simulink model "idq"  (R2021a)
settings: Solver=VariableStepAuto  StartTime=0.0  StopTime=0.2  FixedStep=1/150000  MaxStep=1e-6
undefined symbols (not defined in the file): in, ou
libraries: neural x105, spsMosfetLib x12, simulink x5, pid_lib x3, spsabctodq0Lib x3, spsFirstOrderFilterLib x2, spsPermanentMagnetSynchronousMachineLib x2, spsCurrentMeasurementLib x2, spsDCVoltageSourceLib x2, spsThreePhaseVIMeasurementLib x2, spsabctoAlphaBetaZeroLib x2, spsSVPWMGenerator2LevelLib x1
(part 6 of 7)

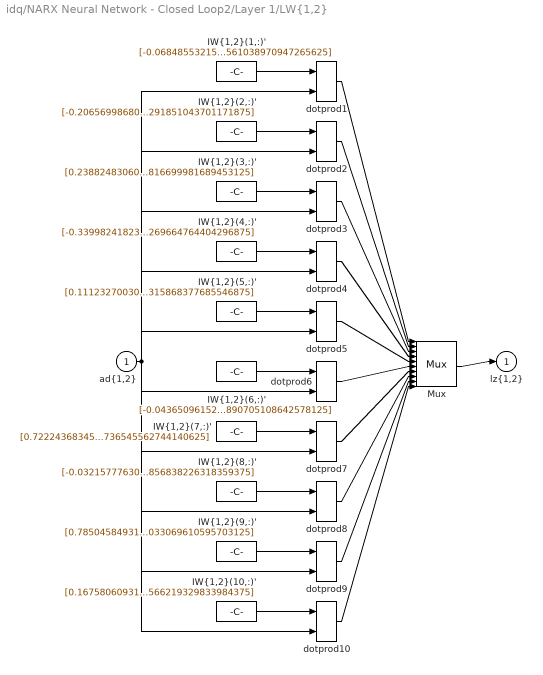
== system idq/NARX Neural Network - Closed Loop2/Layer 1/LW{1,2} ==
  "ad{1,2}" : Inport  PortDimensions=10  SampleTime=1e-05
      mask Display: e = 0.06;c1 = [120 230 180]/255;c2 = ([120 230 180]+0)/(256+128);c3 = ([120 230 180]+128)/(256+128);patch([0 1 1 0],[0 0 1 1],c1);patch([0 1 1 1-e 1-e 0+e],[0 0 1 1-e 0+e 0+e],c2);patch([0 0 1 1-e 0+e 0+e],[0 1 1 1-e 1-e 0+e],c3);plot([0 1 1 0 0],[0 0 1 1 0]);
  "IW{1,2}(1,:)'" : Constant  Value=[-0.06848553215792078929791131258753011934459209442138671875;-0.168183592807916448830241051837219856679439544677734375;-0.0232648098321999417803507270718910149298608303070068359375;0.0222599968251831863141898537605811725370585918426513671875;0.1559933939712914441333424520053085871040821075439453125;0.1043118802673528022761928468753467313945293426513671875;-0.10830870825632206433386528487972100265324115753173828125;-0.06587364865356681864483334720716811716556549072265625;0.1045799553153159144880390840626205317676067352294921875;-0.0238569322650025207599444598827176378108561038970947265625]
      mask Display: e = 0.06;c1 = [120 150 230]/255;c2 = ([120 150 230]+0)/383;c3 = ([120 150 230]+128)/383;patch([0 1 1 0],[0 0 1 1],c1);patch([0 1 1 1-e 1-e 0+e],[0 0 1 1-e 0+e 0+e],c2);patch([0 0 1 1-e 0+e 0+e],[0 1 1 1-e 1-e 0+e],c3);plot([0 1 1 0 0],[0 0 1 1 0]);disp('weights');
  "IW{1,2}(10,:)'" : Constant  Value=[0.167580609319410267499250721812131814658641815185546875;-0.033693308851453822316823760729675996117293834686279296875;-0.02316251894436265057475310413792612962424755096435546875;-0.1505391673267879870667940167550113983452320098876953125;0.0771320191346646921726204482183675281703472137451171875;-0.01480470085334451534053723520401035784743726253509521484375;0.01030379682128204459068410159261475200764834880828857421875;0.0170955227174202674389480449690381647087633609771728515625;-0.1803345239355904905398375603908789344131946563720703125;0.1414515538710732212024367981939576566219329833984375]
      mask Display: e = 0.06;c1 = [120 150 230]/255;c2 = ([120 150 230]+0)/383;c3 = ([120 150 230]+128)/383;patch([0 1 1 0],[0 0 1 1],c1);patch([0 1 1 1-e 1-e 0+e],[0 0 1 1-e 0+e 0+e],c2);patch([0 0 1 1-e 0+e 0+e],[0 1 1 1-e 1-e 0+e],c3);plot([0 1 1 0 0],[0 0 1 1 0]);disp('weights');
  "IW{1,2}(2,:)'" : Constant  Value=[-0.206569986808232075592428600430139340460300445556640625;-0.17704285291305799088235062299645505845546722412109375;0.067029514515075272473865197753184475004673004150390625;-0.11298701828022028603726312212529592216014862060546875;0.44502267784332227851251673200749792158603668212890625;0.0635628244876923209627506139440811239182949066162109375;-0.31596978877279990882698257337324321269989013671875;-0.159523136450386238127663318664417602121829986572265625;-0.026269199652980655679268551239147200249135494232177734375;0.193965717402612980446718893290380947291851043701171875]
      mask Display: e = 0.06;c1 = [120 150 230]/255;c2 = ([120 150 230]+0)/383;c3 = ([120 150 230]+128)/383;patch([0 1 1 0],[0 0 1 1],c1);patch([0 1 1 1-e 1-e 0+e],[0 0 1 1-e 0+e 0+e],c2);patch([0 0 1 1-e 0+e 0+e],[0 1 1 1-e 1-e 0+e],c3);plot([0 1 1 0 0],[0 0 1 1 0]);disp('weights');
  "IW{1,2}(3,:)'" : Constant  Value=[0.2388248306077005722602990545055945403873920440673828125;-0.022260383608824006740345424759652814827859401702880859375;-0.11939523610495351990667955988101311959326267242431640625;-0.1639270891371009952752757499183644540607929229736328125;0.39292260806126522165726555613218806684017181396484375;0.13655922559615196743010301361209712922573089599609375;-0.20158757850580144577179453335702419281005859375;-0.2125949397905498583494221520595601759850978851318359375;0.214255988741538339059644613371347077190876007080078125;0.0736149453097654504762914484672364778816699981689453125]
      mask Display: e = 0.06;c1 = [120 150 230]/255;c2 = ([120 150 230]+0)/383;c3 = ([120 150 230]+128)/383;patch([0 1 1 0],[0 0 1 1],c1);patch([0 1 1 1-e 1-e 0+e],[0 0 1 1-e 0+e 0+e],c2);patch([0 0 1 1-e 0+e 0+e],[0 1 1 1-e 1-e 0+e],c3);plot([0 1 1 0 0],[0 0 1 1 0]);disp('weights');
  "IW{1,2}(4,:)'" : Constant  Value=[-0.339982418230844685158587026307941414415836334228515625;0.06286791591134743839575094170868396759033203125;0.042782434851617374971244345260856789536774158477783203125;0.61568812941807304905950104512157849967479705810546875;-0.484514132046519330199174646622850559651851654052734375;-0.0970863636307574273676124221310601569712162017822265625;0.1572777042332852148742716735796420834958553314208984375;0.20099707904543751002535145744332112371921539306640625;0.235554356615042037592644419419229961931705474853515625;-0.3985764861287808269452170861768536269664764404296875]
      mask Display: e = 0.06;c1 = [120 150 230]/255;c2 = ([120 150 230]+0)/383;c3 = ([120 150 230]+128)/383;patch([0 1 1 0],[0 0 1 1],c1);patch([0 1 1 1-e 1-e 0+e],[0 0 1 1-e 0+e 0+e],c2);patch([0 0 1 1-e 0+e 0+e],[0 1 1 1-e 1-e 0+e],c3);plot([0 1 1 0 0],[0 0 1 1 0]);disp('weights');
  "IW{1,2}(5,:)'" : Constant  Value=[0.11123270030713751366224784078440279699862003326416015625;0.0441165371646720372300620738315046764910221099853515625;0.0337872497512030356414669540754402987658977508544921875;-0.1605454306752725213147670046964776702225208282470703125;0.0023510123039627607577362056190395378507673740386962890625;0.0243052304300900023914522307677543722093105316162109375;0.025135399965839778924081571176429861225187778472900390625;-0.02490004066075475475106060230245930142700672149658203125;-0.03397034171832931381818099225711193867027759552001953125;0.09640861696046380824309807167082908563315868377685546875]
      mask Display: e = 0.06;c1 = [120 150 230]/255;c2 = ([120 150 230]+0)/383;c3 = ([120 150 230]+128)/383;patch([0 1 1 0],[0 0 1 1],c1);patch([0 1 1 1-e 1-e 0+e],[0 0 1 1-e 0+e 0+e],c2);patch([0 0 1 1-e 0+e 0+e],[0 1 1 1-e 1-e 0+e],c3);plot([0 1 1 0 0],[0 0 1 1 0]);disp('weights');
  "IW{1,2}(6,:)'" : Constant  Value=[-0.043650961523407139086572215092019177973270416259765625;-0.0310808465779854707633500510155499796383082866668701171875;0.020776758678725339157811191626024083234369754791259765625;0.00987290351155388490322906136498204432427883148193359375;0.033604488073563969219303970703549566678702831268310546875;-0.05455938140951634152120419685161323286592960357666015625;-0.0510714350539601957823521161117241717875003814697265625;0.045197639986406086543002658117984537966549396514892578125;-0.0495999610894839182417825895754504017531871795654296875;-0.007247288368574862638116229618390207178890705108642578125]
      mask Display: e = 0.06;c1 = [120 150 230]/255;c2 = ([120 150 230]+0)/383;c3 = ([120 150 230]+128)/383;patch([0 1 1 0],[0 0 1 1],c1);patch([0 1 1 1-e 1-e 0+e],[0 0 1 1-e 0+e 0+e],c2);patch([0 0 1 1-e 0+e 0+e],[0 1 1 1-e 1-e 0+e],c3);plot([0 1 1 0 0],[0 0 1 1 0]);disp('weights');
  "IW{1,2}(7,:)'" : Constant  Value=[0.72224368345128520108033853830420412123203277587890625;-0.29672427963986247601013701569172553718090057373046875;-0.5219792424542266662257361531374044716358184814453125;-0.35115714045900736639538308736518956720829010009765625;0.40301906060842485057804651660262607038021087646484375;0.10200757360121469330405119535498670302331447601318359375;-0.03903474384426190713082149841284262947738170623779296875;0.0407956879638946556809742105542682111263275146484375;0.27212331081209339966875404570600949227809906005859375;0.120339102854654600438522038530209101736545562744140625]
      mask Display: e = 0.06;c1 = [120 150 230]/255;c2 = ([120 150 230]+0)/383;c3 = ([120 150 230]+128)/383;patch([0 1 1 0],[0 0 1 1],c1);patch([0 1 1 1-e 1-e 0+e],[0 0 1 1-e 0+e 0+e],c2);patch([0 0 1 1-e 0+e 0+e],[0 1 1 1-e 1-e 0+e],c3);plot([0 1 1 0 0],[0 0 1 1 0]);disp('weights');
  "IW{1,2}(8,:)'" : Constant  Value=[-0.03215777630550940846543284123981720767915248870849609375;-0.15179539790991791736729510375880636274814605712890625;0.044477295640847402946604915996431373059749603271484375;-0.383254418254840578672570927665219642221927642822265625;0.555254658952926138937300493125803768634796142578125;0.4168867115597614247946012255852110683917999267578125;-0.2437911984166573342580619510044925846159458160400390625;-0.6246901165206126815832021748065017163753509521484375;0.72781955521921093410497860531904734671115875244140625;-0.007339261862083799881073531423680833540856838226318359375]
      mask Display: e = 0.06;c1 = [120 150 230]/255;c2 = ([120 150 230]+0)/383;c3 = ([120 150 230]+128)/383;patch([0 1 1 0],[0 0 1 1],c1);patch([0 1 1 1-e 1-e 0+e],[0 0 1 1-e 0+e 0+e],c2);patch([0 0 1 1-e 0+e 0+e],[0 1 1 1-e 1-e 0+e],c3);plot([0 1 1 0 0],[0 0 1 1 0]);disp('weights');
  "IW{1,2}(9,:)'" : Constant  Value=[0.78504584931199727915185349047533236443996429443359375;0.252420705465960681923576203189441002905368804931640625;-0.446249033364787661692929532364360056817531585693359375;0.006236623888100943646772833517388789914548397064208984375;-0.229719455430527019768049967751721851527690887451171875;0.132202063827780824656343838796601630747318267822265625;0.186514759811286179314038236043415963649749755859375;0.1583920339325100845595528653575456701219081878662109375;0.418456055887584332797501929235295392572879791259765625;-0.399445269839285910240533894466352649033069610595703125]
      mask Display: e = 0.06;c1 = [120 150 230]/255;c2 = ([120 150 230]+0)/383;c3 = ([120 150 230]+128)/383;patch([0 1 1 0],[0 0 1 1],c1);patch([0 1 1 1-e 1-e 0+e],[0 0 1 1-e 0+e 0+e],c2);patch([0 0 1 1-e 0+e 0+e],[0 1 1 1-e 1-e 0+e],c3);plot([0 1 1 0 0],[0 0 1 1 0]);disp('weights');
  Mux : Mux  Inputs=10
      mask Display: e = 0.06;c1 = [120 150 230]/255;c2 = ([120 150 230]+0)/383;c3 = ([120 150 230]+128)/383;patch([0 1 1 0],[0 0 1 1],c1);patch([0 1 1 1-e 1-e 0+e],[0 0 1 1-e 0+e 0+e],c2);patch([0 0 1 1-e 0+e 0+e],[0 1 1 1-e 1-e 0+e],c3);plot([0 1 1 0 0],[0 0 1 1 0]);disp('Mux');
  dotprod{1..10} (10 alike) : neural/Weight Functions/dotprod
  "lz{1,2}" : Outport
      mask Display: e = 0.06;c1 = [120 230 180]/255;c2 = ([120 230 180]+0)/(256+128);c3 = ([120 230 180]+128)/(256+128);patch([0 1 1 0],[0 0 1 1],c1);patch([0 1 1 1-e 1-e 0+e],[0 0 1 1-e 0+e 0+e],c2);patch([0 0 1 1-e 0+e 0+e],[0 1 1 1-e 1-e 0+e],c3);plot([0 1 1 0 0],[0 0 1 1 0]);
  wires:
  "IW{1,2}(1,:)'"/1 -> dotprod1/1
  "ad{1,2}"/1 -> dotprod1/2, dotprod2/2, dotprod3/2, dotprod4/2, dotprod5/2, dotprod6/2, dotprod7/2, dotprod8/2, dotprod9/2, dotprod10/2
  dotprod1/1 -> Mux/1
  "IW{1,2}(2,:)'"/1 -> dotprod2/1
  dotprod2/1 -> Mux/2
  "IW{1,2}(3,:)'"/1 -> dotprod3/1
  dotprod3/1 -> Mux/3
  "IW{1,2}(4,:)'"/1 -> dotprod4/1
  dotprod4/1 -> Mux/4
  "IW{1,2}(5,:)'"/1 -> dotprod5/1
  dotprod5/1 -> Mux/5
  "IW{1,2}(6,:)'"/1 -> dotprod6/1
  dotprod6/1 -> Mux/6
  "IW{1,2}(7,:)'"/1 -> dotprod7/1
  dotprod7/1 -> Mux/7
  "IW{1,2}(8,:)'"/1 -> dotprod8/1
  dotprod8/1 -> Mux/8
  "IW{1,2}(9,:)'"/1 -> dotprod9/1
  dotprod9/1 -> Mux/9
  "IW{1,2}(10,:)'"/1 -> dotprod10/1
  dotprod10/1 -> Mux/10
  Mux/1 -> "lz{1,2}"/1

== system idq/NARX Neural Network - Closed Loop2/Layer 2/Delays 1 ==
  "p{2}" : Inport  PortDimensions=10  SampleTime=1e-05
      mask Display: e = 0.06;c1 = [120 230 180]/255;c2 = ([120 230 180]+0)/(256+128);c3 = ([120 230 180]+128)/(256+128);patch([0 1 1 0],[0 0 1 1],c1);patch([0 1 1 1-e 1-e 0+e],[0 0 1 1-e 0+e 0+e],c2);patch([0 0 1 1-e 0+e 0+e],[0 1 1 1-e 1-e 0+e],c3);plot([0 1 1 0 0],[0 0 1 1 0]);
  mux : Mux  Inputs=1
      mask Display: e = 0.06;c1 = [120 150 230]/255;c2 = ([120 150 230]+0)/383;c3 = ([120 150 230]+128)/383;patch([0 1 1 0],[0 0 1 1],c1);patch([0 1 1 1-e 1-e 0+e],[0 0 1 1-e 0+e 0+e],c2);patch([0 0 1 1-e 0+e 0+e],[0 1 1 1-e 1-e 0+e],c3);plot([0 1 1 0 0],[0 0 1 1 0]);disp('Mux')
  "pd{2,1}" : Outport
      mask Display: e = 0.06;c1 = [120 230 180]/255;c2 = ([120 230 180]+0)/(256+128);c3 = ([120 230 180]+128)/(256+128);patch([0 1 1 0],[0 0 1 1],c1);patch([0 1 1 1-e 1-e 0+e],[0 0 1 1-e 0+e 0+e],c2);patch([0 0 1 1-e 0+e 0+e],[0 1 1 1-e 1-e 0+e],c3);plot([0 1 1 0 0],[0 0 1 1 0]);
  wires:
  "p{2}"/1 -> mux/1
  mux/1 -> "pd{2,1}"/1

== system idq/NARX Neural Network - Closed Loop2/Layer 2/LW{2,1} ==
  "ad{2,1}" : Inport  PortDimensions=10  SampleTime=1e-05
      mask Display: e = 0.06;c1 = [120 230 180]/255;c2 = ([120 230 180]+0)/(256+128);c3 = ([120 230 180]+128)/(256+128);patch([0 1 1 0],[0 0 1 1],c1);patch([0 1 1 1-e 1-e 0+e],[0 0 1 1-e 0+e 0+e],c2);patch([0 0 1 1-e 0+e 0+e],[0 1 1 1-e 1-e 0+e],c3);plot([0 1 1 0 0],[0 0 1 1 0]);
  "IW{2,1}(1,:)'" : Constant  Value=[-1.8024487538491762439463172995601780712604522705078125;1.7858415231748401286182570402161218225955963134765625;-1.0516660228917158459438496720395050942897796630859375;-1.321897069778581457200061777257360517978668212890625;2.196982273081371506151526773464865982532501220703125;1.3943035974706512458709539714618586003780364990234375;-0.9205379723976834238641231422661803662776947021484375;1.012472143579025374293678396497853100299835205078125;1.0636810315768301382632898821611888706684112548828125;-2.066348426610085997623400544398464262485504150390625]
      mask Display: e = 0.06;c1 = [120 150 230]/255;c2 = ([120 150 230]+0)/383;c3 = ([120 150 230]+128)/383;patch([0 1 1 0],[0 0 1 1],c1);patch([0 1 1 1-e 1-e 0+e],[0 0 1 1-e 0+e 0+e],c2);patch([0 0 1 1-e 0+e 0+e],[0 1 1 1-e 1-e 0+e],c3);plot([0 1 1 0 0],[0 0 1 1 0]);disp('weights');
  Mux : Mux  Inputs=1
      mask Display: e = 0.06;c1 = [120 150 230]/255;c2 = ([120 150 230]+0)/383;c3 = ([120 150 230]+128)/383;patch([0 1 1 0],[0 0 1 1],c1);patch([0 1 1 1-e 1-e 0+e],[0 0 1 1-e 0+e 0+e],c2);patch([0 0 1 1-e 0+e 0+e],[0 1 1 1-e 1-e 0+e],c3);plot([0 1 1 0 0],[0 0 1 1 0]);disp('Mux');
  dotprod1 : neural/Weight Functions/dotprod
  "lz{2,1}" : Outport
      mask Display: e = 0.06;c1 = [120 230 180]/255;c2 = ([120 230 180]+0)/(256+128);c3 = ([120 230 180]+128)/(256+128);patch([0 1 1 0],[0 0 1 1],c1);patch([0 1 1 1-e 1-e 0+e],[0 0 1 1-e 0+e 0+e],c2);patch([0 0 1 1-e 0+e 0+e],[0 1 1 1-e 1-e 0+e],c3);plot([0 1 1 0 0],[0 0 1 1 0]);
  wires:
  "IW{2,1}(1,:)'"/1 -> dotprod1/1
  "ad{2,1}"/1 -> dotprod1/2
  dotprod1/1 -> Mux/1
  Mux/1 -> "lz{2,1}"/1

== system idq/Time Delay Neural Network1/Layer 1/Delays 1 ==
  "p{1}" : Inport  PortDimensions=4  SampleTime=1e-05
      mask Display: e = 0.06;c1 = [120 230 180]/255;c2 = ([120 230 180]+0)/(256+128);c3 = ([120 230 180]+128)/(256+128);patch([0 1 1 0],[0 0 1 1],c1);patch([0 1 1 1-e 1-e 0+e],[0 0 1 1-e 0+e 0+e],c2);patch([0 0 1 1-e 0+e 0+e],[0 1 1 1-e 1-e 0+e],c3);plot([0 1 1 0 0],[0 0 1 1 0]);
  Delay 1 : UnitDelay  InitialCondition=pi_input_1_delayed_1  SampleTime=1e-05
      mask Display: e = 0.06;c1 = [120 150 230]/255;c2 = ([120 150 230]+0)/383;c3 = ([120 150 230]+128)/383;patch([0 1 1 0],[0 0 1 1],c1);patch([0 1 1 1-e 1-e 0+e],[0 0 1 1-e 0+e 0+e],c2);patch([0 0 1 1-e 0+e 0+e],[0 1 1 1-e 1-e 0+e],c3);plot([0 1 1 0 0],[0 0 1 1 0]);disp('D')
  Delay 10 : UnitDelay  InitialCondition=pi_input_1_delayed_10  SampleTime=1e-05
      mask Display: e = 0.06;c1 = [120 150 230]/255;c2 = ([120 150 230]+0)/383;c3 = ([120 150 230]+128)/383;patch([0 1 1 0],[0 0 1 1],c1);patch([0 1 1 1-e 1-e 0+e],[0 0 1 1-e 0+e 0+e],c2);patch([0 0 1 1-e 0+e 0+e],[0 1 1 1-e 1-e 0+e],c3);plot([0 1 1 0 0],[0 0 1 1 0]);disp('D')
  Delay 2 : UnitDelay  InitialCondition=pi_input_1_delayed_2  SampleTime=1e-05
      mask Display: e = 0.06;c1 = [120 150 230]/255;c2 = ([120 150 230]+0)/383;c3 = ([120 150 230]+128)/383;patch([0 1 1 0],[0 0 1 1],c1);patch([0 1 1 1-e 1-e 0+e],[0 0 1 1-e 0+e 0+e],c2);patch([0 0 1 1-e 0+e 0+e],[0 1 1 1-e 1-e 0+e],c3);plot([0 1 1 0 0],[0 0 1 1 0]);disp('D')
  Delay 3 : UnitDelay  InitialCondition=pi_input_1_delayed_3  SampleTime=1e-05
      mask Display: e = 0.06;c1 = [120 150 230]/255;c2 = ([120 150 230]+0)/383;c3 = ([120 150 230]+128)/383;patch([0 1 1 0],[0 0 1 1],c1);patch([0 1 1 1-e 1-e 0+e],[0 0 1 1-e 0+e 0+e],c2);patch([0 0 1 1-e 0+e 0+e],[0 1 1 1-e 1-e 0+e],c3);plot([0 1 1 0 0],[0 0 1 1 0]);disp('D')
  Delay 4 : UnitDelay  InitialCondition=pi_input_1_delayed_4  SampleTime=1e-05
      mask Display: e = 0.06;c1 = [120 150 230]/255;c2 = ([120 150 230]+0)/383;c3 = ([120 150 230]+128)/383;patch([0 1 1 0],[0 0 1 1],c1);patch([0 1 1 1-e 1-e 0+e],[0 0 1 1-e 0+e 0+e],c2);patch([0 0 1 1-e 0+e 0+e],[0 1 1 1-e 1-e 0+e],c3);plot([0 1 1 0 0],[0 0 1 1 0]);disp('D')
  Delay 5 : UnitDelay  InitialCondition=pi_input_1_delayed_5  SampleTime=1e-05
      mask Display: e = 0.06;c1 = [120 150 230]/255;c2 = ([120 150 230]+0)/383;c3 = ([120 150 230]+128)/383;patch([0 1 1 0],[0 0 1 1],c1);patch([0 1 1 1-e 1-e 0+e],[0 0 1 1-e 0+e 0+e],c2);patch([0 0 1 1-e 0+e 0+e],[0 1 1 1-e 1-e 0+e],c3);plot([0 1 1 0 0],[0 0 1 1 0]);disp('D')
  Delay 6 : UnitDelay  InitialCondition=pi_input_1_delayed_6  SampleTime=1e-05
      mask Display: e = 0.06;c1 = [120 150 230]/255;c2 = ([120 150 230]+0)/383;c3 = ([120 150 230]+128)/383;patch([0 1 1 0],[0 0 1 1],c1);patch([0 1 1 1-e 1-e 0+e],[0 0 1 1-e 0+e 0+e],c2);patch([0 0 1 1-e 0+e 0+e],[0 1 1 1-e 1-e 0+e],c3);plot([0 1 1 0 0],[0 0 1 1 0]);disp('D')
  Delay 7 : UnitDelay  InitialCondition=pi_input_1_delayed_7  SampleTime=1e-05
      mask Display: e = 0.06;c1 = [120 150 230]/255;c2 = ([120 150 230]+0)/383;c3 = ([120 150 230]+128)/383;patch([0 1 1 0],[0 0 1 1],c1);patch([0 1 1 1-e 1-e 0+e],[0 0 1 1-e 0+e 0+e],c2);patch([0 0 1 1-e 0+e 0+e],[0 1 1 1-e 1-e 0+e],c3);plot([0 1 1 0 0],[0 0 1 1 0]);disp('D')
  Delay 8 : UnitDelay  InitialCondition=pi_input_1_delayed_8  SampleTime=1e-05
      mask Display: e = 0.06;c1 = [120 150 230]/255;c2 = ([120 150 230]+0)/383;c3 = ([120 150 230]+128)/383;patch([0 1 1 0],[0 0 1 1],c1);patch([0 1 1 1-e 1-e 0+e],[0 0 1 1-e 0+e 0+e],c2);patch([0 0 1 1-e 0+e 0+e],[0 1 1 1-e 1-e 0+e],c3);plot([0 1 1 0 0],[0 0 1 1 0]);disp('D')
  Delay 9 : UnitDelay  InitialCondition=pi_input_1_delayed_9  SampleTime=1e-05
      mask Display: e = 0.06;c1 = [120 150 230]/255;c2 = ([120 150 230]+0)/383;c3 = ([120 150 230]+128)/383;patch([0 1 1 0],[0 0 1 1],c1);patch([0 1 1 1-e 1-e 0+e],[0 0 1 1-e 0+e 0+e],c2);patch([0 0 1 1-e 0+e 0+e],[0 1 1 1-e 1-e 0+e],c3);plot([0 1 1 0 0],[0 0 1 1 0]);disp('D')
  mux : Mux  Inputs=10
      mask Display: e = 0.06;c1 = [120 150 230]/255;c2 = ([120 150 230]+0)/383;c3 = ([120 150 230]+128)/383;patch([0 1 1 0],[0 0 1 1],c1);patch([0 1 1 1-e 1-e 0+e],[0 0 1 1-e 0+e 0+e],c2);patch([0 0 1 1-e 0+e 0+e],[0 1 1 1-e 1-e 0+e],c3);plot([0 1 1 0 0],[0 0 1 1 0]);disp('Mux')
  "pd{1,1}" : Outport
      mask Display: e = 0.06;c1 = [120 230 180]/255;c2 = ([120 230 180]+0)/(256+128);c3 = ([120 230 180]+128)/(256+128);patch([0 1 1 0],[0 0 1 1],c1);patch([0 1 1 1-e 1-e 0+e],[0 0 1 1-e 0+e 0+e],c2);patch([0 0 1 1-e 0+e 0+e],[0 1 1 1-e 1-e 0+e],c3);plot([0 1 1 0 0],[0 0 1 1 0]);
  wires:
  "p{1}"/1 -> Delay 1/1
  Delay 1/1 -> Delay 2/1, mux/1
  Delay 2/1 -> Delay 3/1, mux/2
  Delay 3/1 -> Delay 4/1, mux/3
  Delay 4/1 -> Delay 5/1, mux/4
  Delay 5/1 -> Delay 6/1, mux/5
  Delay 6/1 -> Delay 7/1, mux/6
  Delay 7/1 -> Delay 8/1, mux/7
  Delay 8/1 -> Delay 9/1, mux/8
  Delay 9/1 -> Delay 10/1, mux/9
  Delay 10/1 -> mux/10
  mux/1 -> "pd{1,1}"/1

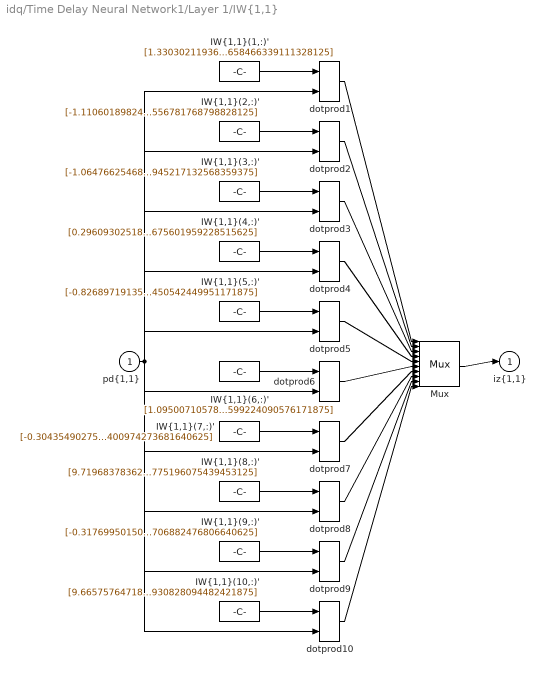
== system idq/Time Delay Neural Network1/Layer 1/IW{1,1} ==
  "pd{1,1}" : Inport  PortDimensions=40  SampleTime=1e-05
      mask Display: e = 0.06;c1 = [120 230 180]/255;c2 = ([120 230 180]+0)/(256+128);c3 = ([120 230 180]+128)/(256+128);patch([0 1 1 0],[0 0 1 1],c1);patch([0 1 1 1-e 1-e 0+e],[0 0 1 1-e 0+e 0+e],c2);patch([0 0 1 1-e 0+e 0+e],[0 1 1 1-e 1-e 0+e],c3);plot([0 1 1 0 0],[0 0 1 1 0]);
  "IW{1,1}(1,:)'" : Constant  Value=[1.330302119368188318304646600154228508472442626953125;0.0926808503977066544532448233439936302602291107177734375;-11.289158332529421358003673958592116832733154296875;10.5997790536904705760434808325953781604766845703125;-0.139965464238469505797723968498758040368556976318359375;-0.93598840560570495394898671293049119412899017333984375;-8.4957112256748370526793223689310252666473388671875;7.4618720824951143555381349870003759860992431640625;2.29448920327525396345436092815361917018890380859375;0.1828678635635263283187867955348338000476360321044921875;-6.07154144858802879980430589057505130767822265625;4.4847061641032386347660576575435698032379150390625;1.1386507448784135565489350483403541147708892822265625;-1.3104699105953994120454808580689132213592529296875;-3.484849633365981080856954577029682695865631103515625;2.53157095435117884818509992328472435474395751953125;0.93594325080031570696093012884375639259815216064453125;1.95238138330620358829037286341190338134765625;-0.9779777814094707810710360718076117336750030517578125;0.1335327171050001704433185523157590068876743316650390625;3.273885083459501910141398184350691735744476318359375;-2.667069712715628870824957630247808992862701416015625;0.70903181136450743604626723026740364730358123779296875;-1.7962124391994842564912460147752426564693450927734375;1.3621955379309544920118923982954584062099456787109375;0.5160216648897499869264038352412171661853790283203125;3.553473278885272090832359026535414159297943115234375;-2.943744115727891852429820573888719081878662109375;2.852745024146873031867244208115153014659881591796875;-1.0748296865231912189386775935417972505092620849609375;5.4310407383714878193359254510141909122467041015625;-4.75849780136871913782670162618160247802734375;-0.450818240941460945947483196505345404148101806640625;1.0479042130998081905346452913363464176654815673828125;7.69703082317251219279796714545227587223052978515625;-6.1095659414790386421145740314386785030364990234375;1.70756109403954337011555253411643207073211669921875;-0.78524162681205178504484365475946106016635894775390625;9.3710390444760012229608037159778177738189697265625;-6.794064690423727626011896063573658466339111328125]
      mask Display: e = 0.06;c1 = [120 150 230]/255;c2 = ([120 150 230]+0)/383;c3 = ([120 150 230]+128)/383;patch([0 1 1 0],[0 0 1 1],c1);patch([0 1 1 1-e 1-e 0+e],[0 0 1 1-e 0+e 0+e],c2);patch([0 0 1 1-e 0+e 0+e],[0 1 1 1-e 1-e 0+e],c3);plot([0 1 1 0 0],[0 0 1 1 0]);disp('Weights');
  "IW{1,1}(10,:)'" : Constant  Value=[9.6657576471839075082925774040631949901580810546875;-0.93242579772732003817736767814494669437408447265625;-18.698426706712009348620995297096669673919677734375;26.779044523422935952794432523660361766815185546875;-2.034124866753716620593195330002345144748687744140625;-3.151479330504836529058820815407671034336090087890625;-16.060776763239829278973047621548175811767578125;16.596927979684547693750573671422898769378662109375;2.038466071333968177015094624948687851428985595703125;-1.801784895016764753705729162902571260929107666015625;-12.5879399133163811796976006007753312587738037109375;7.44556767805154517958499127416871488094329833984375;6.1383369604159039312207823968492448329925537109375;-0.27189923600096188582853073967271484434604644775390625;-9.8053919965394360502841664128936827182769775390625;0.32696013045254701534503283255617134273052215576171875;4.4856747267510730381445682724006474018096923828125;-0.07084793105574270499769085063235252164304256439208984375;-6.05531412554060732844618542003445327281951904296875;-5.09977014294147590334205233375541865825653076171875;6.24565935293380913861938097397796809673309326171875;-5.60269037975893180458797360188327729701995849609375;-1.4289647266589675655978908253018744289875030517578125;-9.244813628891538570542252273298799991607666015625;4.31334923717945084575831060647033154964447021484375;4.089195700832757296439012861810624599456787109375;2.667051680176146799539083076524548232555389404296875;-12.462993725324199800752467126585543155670166015625;3.338572482862902202072064028470776975154876708984375;-3.228402146954106211040880225482396781444549560546875;7.66927642071734538831151439808309078216552734375;-13.68940364740421244960089097730815410614013671875;-0.439376484141544676464974372720462270081043243408203125;2.160465363740531774539022080716677010059356689453125;13.8158554681102661021441235789097845554351806640625;-13.2760374871164348320462522679008543491363525390625;15.369051240367301858213977538980543613433837890625;-0.65745522775927833780684750308864749968051910400390625;19.19887941275109000116572133265435695648193359375;-11.029016063692960614162075216881930828094482421875]
      mask Display: e = 0.06;c1 = [120 150 230]/255;c2 = ([120 150 230]+0)/383;c3 = ([120 150 230]+128)/383;patch([0 1 1 0],[0 0 1 1],c1);patch([0 1 1 1-e 1-e 0+e],[0 0 1 1-e 0+e 0+e],c2);patch([0 0 1 1-e 0+e 0+e],[0 1 1 1-e 1-e 0+e],c3);plot([0 1 1 0 0],[0 0 1 1 0]);disp('Weights');
  "IW{1,1}(2,:)'" : Constant  Value=[-1.11060189824853683404626281117089092731475830078125;-0.634355483276243692358775660977698862552642822265625;8.007935527944255227339453995227813720703125;35.20006104165646121373356436379253864288330078125;1.8694195024596862442223255129647441208362579345703125;-1.7948670344789554587094926318968646228313446044921875;3.305972230423940505517066412721760571002960205078125;23.6973929601222010887795477174222469329833984375;1.3383697797335145640573728087474592030048370361328125;-3.191894435883490199756806759978644549846649169921875;-0.3321857493100186520251781985280103981494903564453125;13.4864167670057906178726625512354075908660888671875;1.25128695648179988353376757004298269748687744140625;-3.737658995654691285182025239919312298297882080078125;-1.892044664519383356804382856353186070919036865234375;5.06746563477815126219638841575942933559417724609375;0.7621852884205029265984876474249176681041717529296875;-4.483496930251288148383537190966308116912841796875;-3.241897099886816846492365584708750247955322265625;-0.98153149430567443456396858891821466386318206787109375;2.38693585513065631431572910514660179615020751953125;-4.96435751757834164976657120860181748867034912109375;-3.101832126068827744092004650156013667583465576171875;-7.0737547766223212164504730026237666606903076171875;1.63245157662784645680176254245452582836151123046875;-1.9899890703486011744871575501747429370880126953125;-3.216789801448802332828336147940717637538909912109375;-11.1933316887101792502789976424537599086761474609375;0.611958552397497523855918188928626477718353271484375;-3.554126189256772594404765186482109129428863525390625;-2.28184221148778210164209667709656059741973876953125;-14.2433869026304051885745138861238956451416015625;2.428085971951865484896870839293114840984344482421875;-0.88734059173318191593438086783862672746181488037109375;-0.159641753007905007333278035730472765862941741943359375;-17.349458990424825088894067448563873767852783203125;-0.434803849957229260336788456697831861674785614013671875;-1.5886351143942294417144012186327017843723297119140625;2.704645334573295034630291411303915083408355712890625;-18.422271577060428171535022556781768798828125]
      mask Display: e = 0.06;c1 = [120 150 230]/255;c2 = ([120 150 230]+0)/383;c3 = ([120 150 230]+128)/383;patch([0 1 1 0],[0 0 1 1],c1);patch([0 1 1 1-e 1-e 0+e],[0 0 1 1-e 0+e 0+e],c2);patch([0 0 1 1-e 0+e 0+e],[0 1 1 1-e 1-e 0+e],c3);plot([0 1 1 0 0],[0 0 1 1 0]);disp('Weights');
  "IW{1,1}(3,:)'" : Constant  Value=[-1.064766254685732604912118404172360897064208984375;-0.62373316260274969113908127837930805981159210205078125;1.0127672344055296260734166935435496270656585693359375;29.31008510520009480160297243855893611907958984375;1.9699010847964959491918079947936348617076873779296875;-1.2641054947258540952503835796960629522800445556640625;2.1971716157158720506004101480357348918914794921875;23.032782625794137487673651776276528835296630859375;1.4793613317169158616337654166272841393947601318359375;-2.717446477889536193828234900138340890407562255859375;2.62125004866138855419421815895475447177886962890625;15.7079649003530494866254230146296322345733642578125;1.4870131666335286713120922286179848015308380126953125;-3.237301937813729324489031569100916385650634765625;1.889494890858188558269148416002281010150909423828125;8.33471967686472936520658549852669239044189453125;0.7381605126569212860232482853461988270282745361328125;-4.56929013900100500222833943553268909454345703125;0.19060160087500310766017719288356602191925048828125;1.1460902254123563892562742694281041622161865234375;2.4077269567361678781480804900638759136199951171875;-4.995935967203880778697566711343824863433837890625;-0.86920682329107401553613954092725180089473724365234375;-4.62949381922912461817531948327086865901947021484375;1.2813487005835793031138791775447316467761993408203125;-2.421904726337425817206394640379585325717926025390625;-1.430287383540993051411760461633093655109405517578125;-10.8248683380386498953384943888522684574127197265625;0.5884325297384227493324715396738611161708831787109375;-3.890420596211094927951990030123852193355560302734375;-2.046411352595792099151594811701215803623199462890625;-14.8590459312216136567030844162218272686004638671875;2.2875566194644907369593056500889360904693603515625;-1.266780847304041390799511646036989986896514892578125;-2.00849341542722026332512541557662189006805419921875;-18.57431897349079719106157426722347736358642578125;-0.754488586252782145180617590085603296756744384765625;-1.8163049133703434989683955791406333446502685546875;-1.8267088880499340319829570944420993328094482421875;-20.609919766659967166333444765768945217132568359375]
      mask Display: e = 0.06;c1 = [120 150 230]/255;c2 = ([120 150 230]+0)/383;c3 = ([120 150 230]+128)/383;patch([0 1 1 0],[0 0 1 1],c1);patch([0 1 1 1-e 1-e 0+e],[0 0 1 1-e 0+e 0+e],c2);patch([0 0 1 1-e 0+e 0+e],[0 1 1 1-e 1-e 0+e],c3);plot([0 1 1 0 0],[0 0 1 1 0]);disp('Weights');
  "IW{1,1}(4,:)'" : Constant  Value=[0.296093025184396230198302646385855041444301605224609375;0.195643831089521658128660419606603682041168212890625;-1.806124142656837960885241045616567134857177734375;2.853766420259329805730885709635913372039794921875;-0.02866708709240960162301092850611894391477108001708984375;-0.301135099802591066353585347314947284758090972900390625;0.05266090988321169008568034541895030997693538665771484375;2.915573076616956971207628157571889460086822509765625;0.47236079983660295145142526962445117533206939697265625;-0.1311523542280391418923812807406648062169551849365234375;1.0685434345837550029756357616861350834369659423828125;2.1112647538899214083585320622660219669342041015625;0.08055112566167292598162674721606890670955181121826171875;-0.46053177519765509106974832320702262222766876220703125;1.5513637462885603301998571623698808252811431884765625;1.102577421213051689363737750682048499584197998046875;0.1997074348530637200038739820229238830506801605224609375;-0.317544716506558299951024082474759779870510101318359375;1.7671359215396644781748136665555648505687713623046875;-0.4717822021696778111987669035443104803562164306640625;0.298124112288542020277049005017033778131008148193359375;-0.784132389337983237709295281092636287212371826171875;1.4924438854115222863327971936087124049663543701171875;-1.271185924629623986703563787159509956836700439453125;-0.2400724777836950318832265338642173446714878082275390625;-0.30828601039668079852873461277340538799762725830078125;1.062923223169097486362488780287094414234161376953125;-1.57355705804146683846056475886143743991851806640625;0.12203540376529586897191848038346506655216217041015625;-0.34140623163763705871787124124239198863506317138671875;0.448098059116362967824187535370583645999431610107421875;-1.9271861494138529113939739545457996428012847900390625;-0.2330820349345734954216169398932834155857563018798828125;-0.460568272720645099926883858643122948706150054931640625;-1.4978922254766449118079663094249553978443145751953125;-1.6512391399970860472734557333751581609249114990234375;-0.07875864165994279908478148399808560498058795928955078125;0.024266803822295034132050517428069724701344966888427734375;-4.166922924213327661391303990967571735382080078125;-1.484184891270258876971865902305580675601959228515625]
      mask Display: e = 0.06;c1 = [120 150 230]/255;c2 = ([120 150 230]+0)/383;c3 = ([120 150 230]+128)/383;patch([0 1 1 0],[0 0 1 1],c1);patch([0 1 1 1-e 1-e 0+e],[0 0 1 1-e 0+e 0+e],c2);patch([0 0 1 1-e 0+e 0+e],[0 1 1 1-e 1-e 0+e],c3);plot([0 1 1 0 0],[0 0 1 1 0]);disp('Weights');
  "IW{1,1}(5,:)'" : Constant  Value=[-0.8268971913586273814189553377218544483184814453125;0.01140683104005511816492202115114196203649044036865234375;4.96494333486332184435241288156248629093170166015625;-38.57243215261362223600372090004384517669677734375;-3.299034237073246611515742188203148543834686279296875;0.80341934756693811348071676547988317906856536865234375;3.97087563452996672452854909352026879787445068359375;-30.09306148308915140887620509602129459381103515625;-2.03755256251952676649352724780328571796417236328125;3.7451216037603245467835222370922565460205078125;3.0479500390159390832423014217056334018707275390625;-22.333811326886600312491282238624989986419677734375;-1.7013927880167047934634183548041619360446929931640625;3.54314067601914661764794800546951591968536376953125;2.03653657483669459082875619060359895229339599609375;-14.495269362889512620995446923188865184783935546875;-1.1178425799121445294304066919721662998199462890625;7.05807110956463201745236801798455417156219482421875;0.83679427684229212847100143335410393774509429931640625;-6.55895788887262920496823426219634711742401123046875;-5.98111365870283417933706004987470805644989013671875;5.51840527337680786246210118406452238559722900390625;-0.1900173442743515739294934974168427288532257080078125;2.368543845515763024422994931228458881378173828125;-1.36683649623848424425887060351669788360595703125;3.173208472528227019893165561370551586151123046875;-1.4771334816846490856079299192060716450214385986328125;10.5985016591895391258049130556173622608184814453125;-6.47595573619689179878378126886673271656036376953125;3.83818664989817914801051301765255630016326904296875;-1.734381089461893399317204966791905462741851806640625;18.857275308612127417973169940523803234100341796875;0.70747471108539794482084062110516242682933807373046875;3.352610268090689071840415635961107909679412841796875;-3.36675760795796197299978302908129990100860595703125;27.7712350706586477144810487516224384307861328125;-2.757241287699461640414710927871055901050567626953125;2.789462530562058617533693904988467693328857421875;-4.12189257934493635815442758030258119106292724609375;36.58395495250612583504334907047450542449951171875]
      mask Display: e = 0.06;c1 = [120 150 230]/255;c2 = ([120 150 230]+0)/383;c3 = ([120 150 230]+128)/383;patch([0 1 1 0],[0 0 1 1],c1);patch([0 1 1 1-e 1-e 0+e],[0 0 1 1-e 0+e 0+e],c2);patch([0 0 1 1-e 0+e 0+e],[0 1 1 1-e 1-e 0+e],c3);plot([0 1 1 0 0],[0 0 1 1 0]);disp('Weights');
  "IW{1,1}(6,:)'" : Constant  Value=[1.095007105788721180061884297174401581287384033203125;0.66010783477611856273625789981451816856861114501953125;-0.1964945138422835857472392717681941576302051544189453125;-20.26239904076813758138086996041238307952880859375;-1.83286473801502847180699973250739276409149169921875;0.69721445401636794603206226383917964994907379150390625;-1.1030199191578748951769739505834877490997314453125;-18.864280239275888817473969538696110248565673828125;-1.1389738089454939373723618700751103460788726806640625;2.060429684697540952953431769856251776218414306640625;-1.378978259410559292774678397108800709247589111328125;-16.00648337529172948734412784688174724578857421875;-1.3702541375721892791261780075728893280029296875;2.369160099346463876912594059831462800502777099609375;-1.697853678847121017270183074288070201873779296875;-13.0151959616841512712426265352405607700347900390625;-0.6546744263959849430278836734942160546779632568359375;4.21974801510947994387379367253743112087249755859375;-2.25613242746991904397191319731064140796661376953125;-9.025525506262201957952129305340349674224853515625;-2.573782201823402004947638488374650478363037109375;4.93155513579513016253486057394184172153472900390625;-1.9409474329615985510599784902296960353851318359375;-3.283085328323494866964438188006170094013214111328125;-1.2274507080044412266062181515735574066638946533203125;2.945546694019860023416867988999001681804656982421875;-1.189329900741680656750531852594576776027679443359375;3.29820677405742213039729904267005622386932373046875;-0.9033053043876384524679679088876582682132720947265625;4.81418729336820394593132732552476227283477783203125;0.5685251307799676911969299908378161489963531494140625;12.2974151606405310843683764687739312648773193359375;-2.5770318055619316766069459845311939716339111328125;2.354139737358234896191788720898330211639404296875;3.31603021826156041385047501535154879093170166015625;22.46787597564775040837048436515033245086669921875;0.69343444849892377224165329607785679399967193603515625;2.66787151019084856073959599598310887813568115234375;6.189666497091451446976861916482448577880859375;34.21859562473434124285631696693599224090576171875]
      mask Display: e = 0.06;c1 = [120 150 230]/255;c2 = ([120 150 230]+0)/383;c3 = ([120 150 230]+128)/383;patch([0 1 1 0],[0 0 1 1],c1);patch([0 1 1 1-e 1-e 0+e],[0 0 1 1-e 0+e 0+e],c2);patch([0 0 1 1-e 0+e 0+e],[0 1 1 1-e 1-e 0+e],c3);plot([0 1 1 0 0],[0 0 1 1 0]);disp('Weights');
  "IW{1,1}(7,:)'" : Constant  Value=[-0.30435490275507348645334104730864055454730987548828125;-0.175226140838568300583943937454023398458957672119140625;-3.830989783239015178395447946968488395214080810546875;-10.8086172579638191137973990407772362232208251953125;0.09640899696338427193875730836225557141005992889404296875;0.86361621810073641025695678763440810143947601318359375;-1.6785002517418592393738663304247893393039703369140625;-4.8700352961557324960040205041877925395965576171875;-0.413991009821180977468202399904839694499969482421875;0.84935339331089476644365277024917304515838623046875;-0.2366703621421859249362995569754275493323802947998046875;0.286677878875738756381252869687159545719623565673828125;0.0038092638796876029418092546308116652653552591800689697265625;1.0309316425522292437477744897478260099887847900390625;1.3449395350383144265293822172679938375949859619140625;2.588584452585664497092921010334976017475128173828125;-0.1354051857569101013911705422287923283874988555908203125;0.57378190153553820795906403873232193291187286376953125;2.20293954852985240933094246429391205310821533203125;4.60285618875339874733754186308942735195159912109375;-0.3082262800728570173447451452375389635562896728515625;0.71912856052151841179664870651322416961193084716796875;2.218455350456900010414074131404049694538116455078125;5.24187455325975282249828524072654545307159423828125;0.15259616509447226917473017238080501556396484375;-0.07000038686649610875090132822151645086705684661865234375;2.020111176464816526987533507053740322589874267578125;4.61222048344841795142201590351760387420654296875;-0.26449973168132523415607693095807917416095733642578125;-0.290883539463778983957809032290242612361907958984375;0.96370849755759124821707928276737220585346221923828125;2.33769288360968996443034484400413930416107177734375;0.03177560837677272098655834042801870964467525482177734375;-0.2249046775102785666877736048263614065945148468017578125;-0.322628646415118958135082039007102139294147491455078125;-0.181887384322719836138304572159540839493274688720703125;-0.06047348834413625306982709162184619344770908355712890625;-0.51978749293458414992841198909445665776729583740234375;-2.59841334944712532006860783440060913562774658203125;-4.43935539699830261639590389677323400974273681640625]
      mask Display: e = 0.06;c1 = [120 150 230]/255;c2 = ([120 150 230]+0)/383;c3 = ([120 150 230]+128)/383;patch([0 1 1 0],[0 0 1 1],c1);patch([0 1 1 1-e 1-e 0+e],[0 0 1 1-e 0+e 0+e],c2);patch([0 0 1 1-e 0+e 0+e],[0 1 1 1-e 1-e 0+e],c3);plot([0 1 1 0 0],[0 0 1 1 0]);disp('Weights');
  "IW{1,1}(8,:)'" : Constant  Value=[9.719683783621778871975038782693445682525634765625;-0.99939425256977398870361639637849293649196624755859375;-21.508392396314551575642326497472822666168212890625;6.751059343599099094035409507341682910919189453125;-2.54965172791211092118146552820689976215362548828125;-1.93401721794126757458798238076269626617431640625;-17.00205485687177286990845459513366222381591796875;9.4542183924202021216842695139348506927490234375;1.549733026066599794745570761733688414096832275390625;-0.286906114907087450571765430140658281743526458740234375;-12.1679645160087321897890433319844305515289306640625;10.725273520927789405732255545444786548614501953125;5.66941384594095776350286541855894029140472412109375;0.9774361223150000999027042780653573572635650634765625;-8.557314405442998150874700513668358325958251953125;9.8630707709220342138678461196832358837127685546875;4.1753289207140458216827028081752359867095947265625;0.64906054656740164165995565781486220657825469970703125;-4.0331121707427399769585463218390941619873046875;7.581198546140694105588409001938998699188232421875;6.256938148150982925699281622655689716339111328125;-5.55761596527076395801714170374907553195953369140625;0.74851766701663879910455534627544693648815155029296875;3.838650906612026236786050503724254667758941650390625;4.54008214687524525032813471625559031963348388671875;3.313947521276887631103136300225742161273956298828125;4.67205728505815809370460556237958371639251708984375;-2.666518942882244669334568243357352912425994873046875;3.758295050522805436088447095244191586971282958984375;-4.50381723306763515068951164721511304378509521484375;8.810927852031635865159842069260776042938232421875;-9.51325464560525091428644373081624507904052734375;0.0947147320354703448064270787654095329344272613525390625;0.62669383479237106282511149402125738561153411865234375;12.1809076736155983411435954621993005275726318359375;-19.0044096065721390687031089328229427337646484375;15.6608453227340955749014028697274625301361083984375;-1.831273807752513693714035980519838631153106689453125;15.7769991976055887761276608216576278209686279296875;-30.73272867824852738749541458673775196075439453125]
      mask Display: e = 0.06;c1 = [120 150 230]/255;c2 = ([120 150 230]+0)/383;c3 = ([120 150 230]+128)/383;patch([0 1 1 0],[0 0 1 1],c1);patch([0 1 1 1-e 1-e 0+e],[0 0 1 1-e 0+e 0+e],c2);patch([0 0 1 1-e 0+e 0+e],[0 1 1 1-e 1-e 0+e],c3);plot([0 1 1 0 0],[0 0 1 1 0]);disp('Weights');
  "IW{1,1}(9,:)'" : Constant  Value=[-0.31769950150010217715390581361134536564350128173828125;-0.2206697089816118673155642682104371488094329833984375;-5.1000183370434175600394155480898916721343994140625;2.778057633096675527184515885892324149608612060546875;0.50135844421588393604594102725968696177005767822265625;0.2347061150152629782628110888254013843834400177001953125;-2.1985717739677763660210985108278691768646240234375;-0.323778500725742712784693821959081105887889862060546875;0.1623173482215362339875497355023981072008609771728515625;-0.0305060028100461073929938748960921657271683216094970703125;-0.75404764810586322187901942015741951763629913330078125;-2.5838956934997501235784511663950979709625244140625;0.53066734855448716157155786277144216001033782958984375;0.29381076822161589223725286501576192677021026611328125;1.2981667738393787292494607754633761942386627197265625;-3.886040809534701434557746324571780860424041748046875;0.1815987654296187248093019661610014736652374267578125;0.253693348932645779125749641025322489440441131591796875;1.9630258393386352810949802005779929459095001220703125;-3.8826193233296191209547032485716044902801513671875;-0.2439007161529337663896654930795193649828433990478515625;0.83210555493770088641980464672087691724300384521484375;2.611537520875148121746178730973042547702789306640625;-3.50846633905133398201314776088111102581024169921875;0.01532214087729925899861171956217731349170207977294921875;0.45084359935716111777992409770376980304718017578125;2.681978649233971889742633720743469893932342529296875;-2.4723726448488303475414795684628188610076904296875;-0.65737033030486424767246944611542858183383941650390625;0.6352407466328251484100064772064797580242156982421875;1.4654054062578294459484595790854655206203460693359375;0.42510833735216280171442804203252308070659637451171875;-0.406994241537823153720410118694417178630828857421875;0.74820896576085316187487705974490381777286529541015625;0.10925867060539283526221510101095191203057765960693359375;4.22403088446423691237896491657011210918426513671875;-0.436428371446656360177485112217254936695098876953125;0.1398689996598636298141826728169689886271953582763671875;-2.11182302504321040004242604481987655162811279296875;8.582218840973556694962098845280706882476806640625]
      mask Display: e = 0.06;c1 = [120 150 230]/255;c2 = ([120 150 230]+0)/383;c3 = ([120 150 230]+128)/383;patch([0 1 1 0],[0 0 1 1],c1);patch([0 1 1 1-e 1-e 0+e],[0 0 1 1-e 0+e 0+e],c2);patch([0 0 1 1-e 0+e 0+e],[0 1 1 1-e 1-e 0+e],c3);plot([0 1 1 0 0],[0 0 1 1 0]);disp('Weights');
  Mux : Mux  Inputs=10
      mask Display: e = 0.06;c1 = [120 150 230]/255;c2 = ([120 150 230]+0)/383;c3 = ([120 150 230]+128)/383;patch([0 1 1 0],[0 0 1 1],c1);patch([0 1 1 1-e 1-e 0+e],[0 0 1 1-e 0+e 0+e],c2);patch([0 0 1 1-e 0+e 0+e],[0 1 1 1-e 1-e 0+e],c3);plot([0 1 1 0 0],[0 0 1 1 0]);disp('Mux');
  dotprod{1..10} (10 alike) : neural/Weight Functions/dotprod
  "iz{1,1}" : Outport
      mask Display: e = 0.06;c1 = [120 230 180]/255;c2 = ([120 230 180]+0)/(256+128);c3 = ([120 230 180]+128)/(256+128);patch([0 1 1 0],[0 0 1 1],c1);patch([0 1 1 1-e 1-e 0+e],[0 0 1 1-e 0+e 0+e],c2);patch([0 0 1 1-e 0+e 0+e],[0 1 1 1-e 1-e 0+e],c3);plot([0 1 1 0 0],[0 0 1 1 0]);
  wires:
  "IW{1,1}(1,:)'"/1 -> dotprod1/1
  "pd{1,1}"/1 -> dotprod1/2, dotprod2/2, dotprod3/2, dotprod4/2, dotprod5/2, dotprod6/2, dotprod7/2, dotprod8/2, dotprod9/2, dotprod10/2
  dotprod1/1 -> Mux/1
  "IW{1,1}(2,:)'"/1 -> dotprod2/1
  dotprod2/1 -> Mux/2
  "IW{1,1}(3,:)'"/1 -> dotprod3/1
  dotprod3/1 -> Mux/3
  "IW{1,1}(4,:)'"/1 -> dotprod4/1
  dotprod4/1 -> Mux/4
  "IW{1,1}(5,:)'"/1 -> dotprod5/1
  dotprod5/1 -> Mux/5
  "IW{1,1}(6,:)'"/1 -> dotprod6/1
  dotprod6/1 -> Mux/6
  "IW{1,1}(7,:)'"/1 -> dotprod7/1
  dotprod7/1 -> Mux/7
  "IW{1,1}(8,:)'"/1 -> dotprod8/1
  dotprod8/1 -> Mux/8
  "IW{1,1}(9,:)'"/1 -> dotprod9/1
  dotprod9/1 -> Mux/9
  "IW{1,1}(10,:)'"/1 -> dotprod10/1
  dotprod10/1 -> Mux/10
  Mux/1 -> "iz{1,1}"/1

== system idq/Time Delay Neural Network1/Layer 2/Delays 1 ==
  "p{2}" : Inport  PortDimensions=10  SampleTime=1e-05
      mask Display: e = 0.06;c1 = [120 230 180]/255;c2 = ([120 230 180]+0)/(256+128);c3 = ([120 230 180]+128)/(256+128);patch([0 1 1 0],[0 0 1 1],c1);patch([0 1 1 1-e 1-e 0+e],[0 0 1 1-e 0+e 0+e],c2);patch([0 0 1 1-e 0+e 0+e],[0 1 1 1-e 1-e 0+e],c3);plot([0 1 1 0 0],[0 0 1 1 0]);
  mux : Mux  Inputs=1
      mask Display: e = 0.06;c1 = [120 150 230]/255;c2 = ([120 150 230]+0)/383;c3 = ([120 150 230]+128)/383;patch([0 1 1 0],[0 0 1 1],c1);patch([0 1 1 1-e 1-e 0+e],[0 0 1 1-e 0+e 0+e],c2);patch([0 0 1 1-e 0+e 0+e],[0 1 1 1-e 1-e 0+e],c3);plot([0 1 1 0 0],[0 0 1 1 0]);disp('Mux')
  "pd{2,1}" : Outport
      mask Display: e = 0.06;c1 = [120 230 180]/255;c2 = ([120 230 180]+0)/(256+128);c3 = ([120 230 180]+128)/(256+128);patch([0 1 1 0],[0 0 1 1],c1);patch([0 1 1 1-e 1-e 0+e],[0 0 1 1-e 0+e 0+e],c2);patch([0 0 1 1-e 0+e 0+e],[0 1 1 1-e 1-e 0+e],c3);plot([0 1 1 0 0],[0 0 1 1 0]);
  wires:
  "p{2}"/1 -> mux/1
  mux/1 -> "pd{2,1}"/1

== system idq/Time Delay Neural Network1/Layer 2/LW{2,1} ==
  "ad{2,1}" : Inport  PortDimensions=10  SampleTime=1e-05
      mask Display: e = 0.06;c1 = [120 230 180]/255;c2 = ([120 230 180]+0)/(256+128);c3 = ([120 230 180]+128)/(256+128);patch([0 1 1 0],[0 0 1 1],c1);patch([0 1 1 1-e 1-e 0+e],[0 0 1 1-e 0+e 0+e],c2);patch([0 0 1 1-e 0+e 0+e],[0 1 1 1-e 1-e 0+e],c3);plot([0 1 1 0 0],[0 0 1 1 0]);
  "IW{2,1}(1,:)'" : Constant  Value=[0.1600337908961007304942114615187165327370166778564453125;-11.227275013761580879645407549105584621429443359375;26.741126723657888675234062247909605503082275390625;14.3399449941633836402843371615745127201080322265625;-0.254646384696810834658009525810484774410724639892578125;15.133810834254230570650179288350045680999755859375;8.4349719489586494347577172447927296161651611328125;19.45929383748998731107349158264696598052978515625;6.2014728487652863719858942204155027866363525390625;-19.4090543887832183145292219705879688262939453125]
      mask Display: e = 0.06;c1 = [120 150 230]/255;c2 = ([120 150 230]+0)/383;c3 = ([120 150 230]+128)/383;patch([0 1 1 0],[0 0 1 1],c1);patch([0 1 1 1-e 1-e 0+e],[0 0 1 1-e 0+e 0+e],c2);patch([0 0 1 1-e 0+e 0+e],[0 1 1 1-e 1-e 0+e],c3);plot([0 1 1 0 0],[0 0 1 1 0]);disp('weights');
  Mux : Mux  Inputs=1
      mask Display: e = 0.06;c1 = [120 150 230]/255;c2 = ([120 150 230]+0)/383;c3 = ([120 150 230]+128)/383;patch([0 1 1 0],[0 0 1 1],c1);patch([0 1 1 1-e 1-e 0+e],[0 0 1 1-e 0+e 0+e],c2);patch([0 0 1 1-e 0+e 0+e],[0 1 1 1-e 1-e 0+e],c3);plot([0 1 1 0 0],[0 0 1 1 0]);disp('Mux');
  dotprod1 : neural/Weight Functions/dotprod
  "lz{2,1}" : Outport
      mask Display: e = 0.06;c1 = [120 230 180]/255;c2 = ([120 230 180]+0)/(256+128);c3 = ([120 230 180]+128)/(256+128);patch([0 1 1 0],[0 0 1 1],c1);patch([0 1 1 1-e 1-e 0+e],[0 0 1 1-e 0+e 0+e],c2);patch([0 0 1 1-e 0+e 0+e],[0 1 1 1-e 1-e 0+e],c3);plot([0 1 1 0 0],[0 0 1 1 0]);
  wires:
  "IW{2,1}(1,:)'"/1 -> dotprod1/1
  "ad{2,1}"/1 -> dotprod1/2
  dotprod1/1 -> Mux/1
  Mux/1 -> "lz{2,1}"/1
